simulink library "vehicle000_cl"  (R2018b)
settings: Solver=VariableStepAuto  StartTime=0.0  StopTime=10.0  RelTol=1e-3
undefined symbols (not defined in the file): simParam, vhcl
libraries: vrlib x1, dragTurbine_ul x1, fluidDynamicSurface_cl x1, fuselage_cl x1, getFluidDynamicCenters_ul x1, sixDoFDynamics_cl x1, tethersMoment_cl x1, thrAttachPtKinematics_ul x1
settings Model: Creator=mcobb  LastModifiedBy=jldanie5

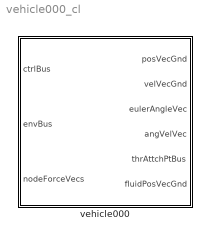
== system vehicle000_cl ==
  vehicle000 : Subsystem  VariantControl=VSS_vehicle_vehicle000  mask{vcl=vhcl, rho=simParam.env_param.density.Value, grav=1}
      mask prompts: vcl "Vehicle"; rho "Density"; grav "Gravity"
      mask DialogControl Container9 Prompt: General
      mask DialogControl Container5 Prompt: Vehicle object (OCT.vehicle)
      mask DialogControl ParameterGroupVar Prompt: Environment Object (OCT.env)
      mask Display:
      | image('kite.jpg',[100 100 601 528]/4,'on')
      | 
      | port_label('input',1,'ctrlBus')
      | port_label('input',2,'envBus')
      | port_label('input',3,'nodeForceVecs')
      | 
      | port_label('output',1,'posVecGnd')
      | port_label('output',2,'velVecGnd')
      | port_label('output',3,'eulAng')
      | port_label('output',4,'angVelVec')
      | port_label('output',5,'thrAttchPtBus')
      | port_label('output',6,'fluidPosVecGnd')

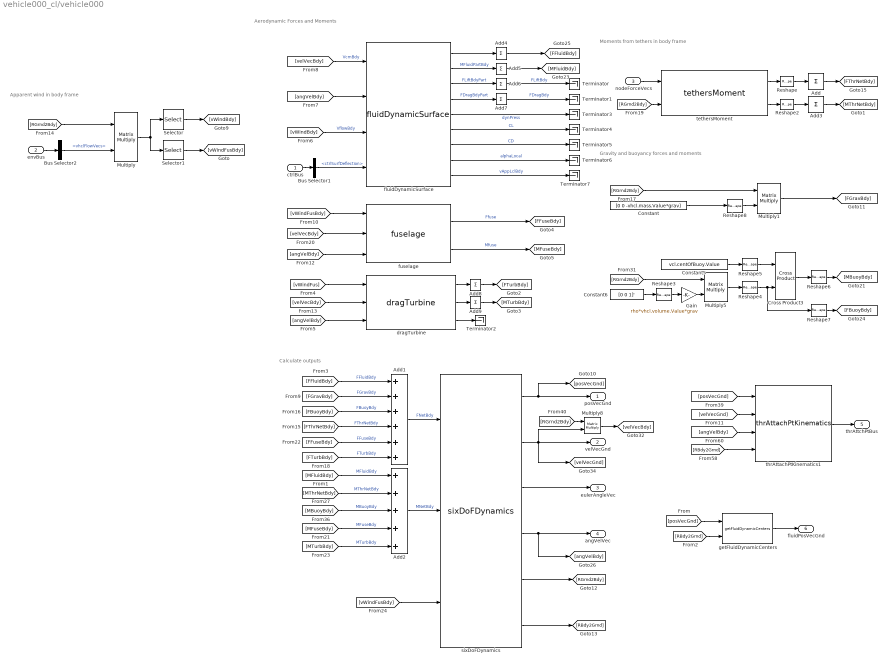
== system vehicle000_cl/vehicle000 ==
  note: Calculate outputs
  note: Apparent wind in body frame
  note: Gravity and buoyancy forces and moments
  note: Moments from tethers in body frame
  note: Aerodynamic Forces and Moments
  ctrlBus : Inport  OutDataTypeStr=Bus: fltCtrlBus
  envBus : Inport  Port=2  OutDataTypeStr=Bus: envBus
  nodeForceVecs : Inport  Port=3
  Add : Sum  Inputs=+  CollapseMode=Specified dimension  CollapseDim=2
  Add1 : Sum  Inputs=++++++
  Add2 : Sum  Inputs=+++++
  Add3 : Sum  Inputs=+  CollapseMode=Specified dimension  CollapseDim=2
  Add{4..9} (6 alike) : Sum  Inputs=1  CollapseMode=Specified dimension  CollapseDim=2
  Bus Selector1 : BusSelector  OutputSignals=ctrlSurfDeflection
  Bus Selector2 : BusSelector  OutputSignals=vhclFlowVecs
  Constant : Constant  Value=[0 0 -vhcl.mass.Value*grav]
  Constant5 : Constant  Value=vcl.centOfBuoy.Value
  Constant6 : Constant  Value=[0 0 1]'
  Cross Product3 : vrlib/Utilities/Cross Product
      settings: SourceProductBaseCode=VR
  Gain : Gain  Gain=rho*vhcl.volume.Value*grav
  Multiply{,1,5,8} (4 alike) : Product  Multiplication=Matrix(*)
  Reshape : Reshape  OutputDimensionality=Customize  OutputDimensions=[3 vcl.numTethers.Value]
  Reshape2 : Reshape  OutputDimensionality=Customize  OutputDimensions=[3 vcl.numTethers.Value]
  Reshape{3..8} (6 alike) : Reshape  OutputDimensionality=Column vector (2-D)
  Selector : Selector  NumberOfDimensions=2  InputPortWidth=3  IndexOptions=Select all,Index vector (dialog)  Indices=[1 3],1:4  OutputSizes=1,1
  Selector1 : Selector  NumberOfDimensions=2  InputPortWidth=3  IndexOptions=Select all,Index vector (dialog)  Indices=[1 3],5  OutputSizes=1,1
  Terminator{,1..7} (8 alike) : Terminator
  dragTurbine : dragTurbine_ul/dragTurbine  rho_fluid=rho  turb_struct=vcl.struct('OCT.turb')
  fluidDynamicSurface : fluidDynamicSurface_cl/fluidDynamicSurface  aeroStruct=vcl.struct('OCT.aeroSurf')  fluidDensity=env.water.density.Value
  fuselage : fuselage_cl/fuselage  fus=vcl.fuse  fusRhoDa=rho
  getFluidDynamicCenters : getFluidDynamicCenters_ul/getFluidDynamicCenters  vcl=vcl
  sixDoFDynamics : sixDoFDynamics_cl/sixDoFDynamics  vcl=vcl
  tethersMoment : tethersMoment_cl/tethersMoment  arms=vcl.struct('OCT.thrAttch')
  thrAttachPtKinematics1 : thrAttachPtKinematics_ul/thrAttachPtKinematics  atchPts=vcl.struct('OCT.thrAttch')
  posVecGnd : Outport
  velVecGnd : Outport  Port=2
  eulerAngleVec : Outport  Port=3
  angVelVec : Outport  Port=4
  thrAttchPtBus : Outport  Port=5
  fluidPosVecGnd : Outport  Port=6
  wires:
  [RGrnd2Bdy] -> Multiply/1
  Multiply/1 -> Selector1/1, Selector/1
  [RGrnd2Bdy] -> Multiply1/1
  Multiply1/1 -> [FGravBdy]
  nodeForceVecs/1 -> tethersMoment/1
  Multiply5/1 -> Reshape4/1
  [RGrnd2Bdy] -> Multiply5/1
  Cross Product3/1 -> Reshape6/1
  Constant5/1 -> Reshape5/1
  [MFluidBdy] -> Add2/1  "MFluidBdy"
  [MThrNetBdy] -> Add2/2  "MThrNetBdy"
  Add2/1 -> sixDoFDynamics/2  "MNetBdy"
  sixDoFDynamics/3 -> eulerAngleVec/1
  sixDoFDynamics/4 -> angVelVec/1, [angVelBdy]
  [FFluidBdy] -> Add1/1  "FFluidBdy"
  Constant/1 -> Reshape8/1
  fluidDynamicSurface/2 -> Add5/1  "MFluidPartBdy"
  sixDoFDynamics/1 -> [posVecGnd], posVecGnd/1
  Multiply8/1 -> [velVecBdy]
  sixDoFDynamics/2 -> [velVecGnd], velVecGnd/1, Multiply8/2
  [RGrnd2Bdy] -> Multiply8/1
  [angVelBdy] -> thrAttachPtKinematics1/3
  thrAttachPtKinematics1/1 -> thrAttchPtBus/1
  [posVecGnd] -> thrAttachPtKinematics1/1
  [RBdy2Grnd] -> thrAttachPtKinematics1/4
  [velVecGnd] -> thrAttachPtKinematics1/2
  tethersMoment/1 -> Reshape/1
  Reshape/1 -> Add/1
  Add/1 -> [FThrNetBdy]
  [RGrnd2Bdy] -> tethersMoment/2
  Bus Selector2/1 -> Multiply/2  "<vhclFlowVecs>"
  Add3/1 -> [MThrNetBdy]
  Reshape2/1 -> Add3/1
  tethersMoment/2 -> Reshape2/1
  Add1/1 -> sixDoFDynamics/1  "FNetBdy"
  envBus/1 -> Bus Selector2/1
  ctrlBus/1 -> Bus Selector1/1
  fluidDynamicSurface/1 -> Add4/1
  fluidDynamicSurface/3 -> Add6/1  "FLiftBdyPart"
  fluidDynamicSurface/4 -> Add7/1  "FDragBdyPart"
  [vWindBdy] -> fluidDynamicSurface/3  "VflowBdy"
  [angVelBdy] -> fluidDynamicSurface/2
  [velVecBdy] -> fluidDynamicSurface/1  "VcmBdy"
  Bus Selector1/1 -> fluidDynamicSurface/4  "<ctrlSurfDeflection>"
  Add4/1 -> [FFluidBdy]
  Add5/1 -> [MFluidBdy]
  Add6/1 -> Terminator/1  "FLiftBdy"
  Add7/1 -> Terminator1/1  "FDragBdy"
  [MBuoyBdy] -> Add2/3  "MBuoyBdy"
  [FThrNetBdy] -> Add1/4  "FThrNetBdy"
  [FBuoyBdy] -> Add1/3  "FBuoyBdy"
  [FGravBdy] -> Add1/2  "FGravBdy"
  Gain/1 -> Multiply5/2
  fluidDynamicSurface/5 -> Terminator3/1  "dynPress"
  fluidDynamicSurface/7 -> Terminator5/1  "CD"
  fluidDynamicSurface/6 -> Terminator4/1  "CL"
  fluidDynamicSurface/8 -> Terminator6/1  "alphaLocal"
  Constant6/1 -> Reshape3/1
  Reshape3/1 -> Gain/1
  Reshape4/1 -> Cross Product3/2, Reshape7/1
  Reshape5/1 -> Cross Product3/1
  Reshape6/1 -> [MBuoyBdy]
  Reshape7/1 -> [FBuoyBdy]
  Reshape8/1 -> Multiply1/2
  [angVelBdy] -> fuselage/3
  [velVecBdy] -> fuselage/2
  [vWindFusBdy] -> fuselage/1
  fuselage/2 -> [MFuseBdy]  "Mfuse"
  fuselage/1 -> [FFuseBdy]  "Ffuse"
  fluidDynamicSurface/9 -> Terminator7/1  "vAppLclBdy"
  [MFuseBdy] -> Add2/4  "MFuseBdy"
  sixDoFDynamics/6 -> [RBdy2Grnd]
  sixDoFDynamics/5 -> [RGrnd2Bdy]
  getFluidDynamicCenters/1 -> fluidPosVecGnd/1
  [FFuseBdy] -> Add1/5  "FFuseBdy"
  Selector/1 -> [vWindBdy]
  Selector1/1 -> [vWindFusBdy]
  [RBdy2Grnd] -> getFluidDynamicCenters/2
  [posVecGnd] -> getFluidDynamicCenters/1
  [vWindFus] -> dragTurbine/1
  [velVecBdy] -> dragTurbine/2
  [angVelBdy] -> dragTurbine/3
  dragTurbine/3 -> Terminator2/1
  dragTurbine/1 -> Add8/1
  dragTurbine/2 -> Add9/1
  [FTurbBdy] -> Add1/6  "FTurbBdy"
  [MTurbBdy] -> Add2/5  "MTurbBdy"
  Add8/1 -> [FTurbBdy]
  Add9/1 -> [MTurbBdy]
  [vWindFusBdy] -> sixDoFDynamics/3
